simulink model "gm_IP_Core_SS_Switch_and_PWM"  (R2021a)
settings: Solver=VariableStepAuto  StartTime=0.0  StopTime=0.001  RelTol=1e-3
undefined symbols (not defined in the file or in its folder): f_FPGA_clk, T_FPGA_clk
libraries: hdlmdlgenlib x3, hdlsllib x3, simulink x2
(part 3 of 3)

== system gm_IP_Core_SS_Switch_and_PWM/PWM_and_Switching_Signal_Control/GenPWM/Triangle shift1/Subsystem1 ==
  standardized peak of triangle : Inport  OutDataTypeStr=fixdt(0, 21, 17)  PortDimensions=1  SampleTime=1e-08
  triangle_in : Inport  Port=2  OutDataTypeStr=fixdt(1, 20, 17)  PortDimensions=1  SampleTime=1e-08
  converted triangle_shift : Inport  Port=3  OutDataTypeStr=fixdt(1, 20, 17)  PortDimensions=1  SampleTime=1e-08
  modified triangle_shift : Inport  Port=4  OutDataTypeStr=fixdt(1, 20, 17)  PortDimensions=1  SampleTime=1e-08
  Zero_input : Inport  Port=5  OutDataTypeStr=boolean  PortDimensions=1  SampleTime=1e-08
  direction up : Inport  Port=6  OutDataTypeStr=boolean  PortDimensions=1  SampleTime=1e-08
  Relational Operator2 : RelationalOperator  OutDataTypeStr=boolean  SampleTime=1e-08  RndMeth=Nearest
  Sum11_stage2 : Sum  AccumDataTypeStr=fixdt(1, 24, 17)  OutDataTypeStr=fixdt(1, 24, 17)  SampleTime=1e-08
  Sum11_stage3 : Sum  Inputs=+-  AccumDataTypeStr=fixdt(1, 24, 17)  OutDataTypeStr=fixdt(1, 21, 17)  SampleTime=1e-08
  Sum6 : Sum  AccumDataTypeStr=fixdt(1, 23, 17)  OutDataTypeStr=fixdt(1, 23, 17)  SampleTime=1e-08
  and1_1 : Switch  Criteria=u2 > Threshold  Threshold=double(0)  OutDataTypeStr=boolean  SampleTime=1e-08
  and1_2 : Switch  Criteria=u2 > Threshold  Threshold=double(0)  OutDataTypeStr=boolean  SampleTime=1e-08
  delayMatch{,1..3} (4 alike) : Delay  DelayLength=double(1)  InitialCondition=0  SampleTime=1e-08
  shifted triangle_in signal : Outport  SampleTime=1e-08
  enable_out : Outport  Port=2  SampleTime=1e-08
  wires:
  delayMatch/1 -> Sum6/2
  delayMatch2/1 -> and1_1/3
  Relational Operator2/1 -> and1_1/2
  Sum11_stage3/1 -> shifted triangle_in signal/1
  Sum6/1 -> Sum11_stage2/2, Relational Operator2/2
  and1_1/1 -> and1_2/1
  and1_2/1 -> enable_out/1
  Sum11_stage2/1 -> Sum11_stage3/1
  standardized peak of triangle/1 -> delayMatch1/1, delayMatch/1
  triangle_in/1 -> Sum11_stage3/2, Relational Operator2/1
  converted triangle_shift/1 -> and1_1/1
  modified triangle_shift/1 -> Sum6/1
  Zero_input/1 -> delayMatch3/1, delayMatch2/1
  direction up/1 -> and1_2/2
  delayMatch1/1 -> Sum11_stage2/1
  delayMatch3/1 -> and1_2/3

== system gm_IP_Core_SS_Switch_and_PWM/PWM_and_Switching_Signal_Control/GenPWM/Triangle shift1/Subsystem2 ==
  triangle_in : Inport  OutDataTypeStr=fixdt(1, 20, 17)  PortDimensions=1  SampleTime=1e-08
  modified triangle_shift : Inport  Port=2  OutDataTypeStr=fixdt(1, 20, 17)  PortDimensions=1  SampleTime=1e-08
  standardized peak of triangle : Inport  Port=3  OutDataTypeStr=fixdt(0, 21, 17)  PortDimensions=1  SampleTime=1e-08
  Zero_input : Inport  Port=4  OutDataTypeStr=boolean  PortDimensions=1  SampleTime=1e-08
  direction down : Inport  Port=5  OutDataTypeStr=boolean  PortDimensions=1  SampleTime=1e-08
  Relational Operator9 : RelationalOperator  OutDataTypeStr=boolean  SampleTime=1e-08  RndMeth=Nearest
  Sum1 : Sum  Inputs=+-  AccumDataTypeStr=fixdt(1, 23, 17)  OutDataTypeStr=fixdt(1, 23, 17)  SampleTime=1e-08
  Sum5_stage2 : Sum  AccumDataTypeStr=fixdt(1, 24, 17)  OutDataTypeStr=fixdt(1, 24, 17)  SampleTime=1e-08
  Sum5_stage3 : Sum  Inputs=+-  AccumDataTypeStr=fixdt(1, 24, 17)  OutDataTypeStr=fixdt(1, 21, 17)  SampleTime=1e-08
  and : Switch  Criteria=u2 > Threshold  Threshold=double(0)  OutDataTypeStr=boolean  SampleTime=1e-08
  delayMatch : Delay  DelayLength=double(1)  InitialCondition=0  SampleTime=1e-08
  delayMatch1 : Delay  DelayLength=double(1)  InitialCondition=0  SampleTime=1e-08
  delayMatch2 : Delay  DelayLength=double(1)  InitialCondition=0  SampleTime=1e-08
  shifted triangle_in signal : Outport  SampleTime=1e-08
  enable_out : Outport  Port=2  SampleTime=1e-08
  wires:
  delayMatch/1 -> Sum1/1
  delayMatch2/1 -> and/3
  Relational Operator9/1 -> and/1
  Sum1/1 -> Sum5_stage2/1, Relational Operator9/2
  Sum5_stage3/1 -> shifted triangle_in signal/1
  and/1 -> enable_out/1
  Sum5_stage2/1 -> Sum5_stage3/1
  triangle_in/1 -> Sum5_stage3/2, Relational Operator9/1
  modified triangle_shift/1 -> Sum1/2
  standardized peak of triangle/1 -> delayMatch1/1, delayMatch/1
  Zero_input/1 -> delayMatch2/1
  direction down/1 -> and/2
  delayMatch1/1 -> Sum5_stage2/2

== system gm_IP_Core_SS_Switch_and_PWM/PWM_and_Switching_Signal_Control/GenPWM/Triangle shift1/Subsystem3 ==
  triangle_in : Inport  OutDataTypeStr=fixdt(1, 20, 17)  PortDimensions=1  SampleTime=1e-08
  modified triangle_shift : Inport  Port=2  OutDataTypeStr=fixdt(1, 20, 17)  PortDimensions=1  SampleTime=1e-08
  direction up : Inport  Port=3  OutDataTypeStr=boolean  PortDimensions=1  SampleTime=1e-08
  Relational Operator6 : RelationalOperator  Operator=<=  OutDataTypeStr=boolean  SampleTime=1e-08  RndMeth=Nearest
  Sum2 : Sum  Inputs=+-  AccumDataTypeStr=fixdt(1, 21, 17)  OutDataTypeStr=fixdt(1, 21, 17)  SampleTime=1e-08
  Sum3 : Sum  Inputs=+-  AccumDataTypeStr=fixdt(1, 21, 17)  OutDataTypeStr=fixdt(1, 21, 17)  SampleTime=1e-08
  Sum4 : Sum  AccumDataTypeStr=fixdt(1, 21, 17)  OutDataTypeStr=fixdt(1, 21, 17)  SampleTime=1e-08
  Switch3 : Switch  Criteria=u2 > Threshold  Threshold=double(0)  OutDataTypeStr=fixdt(1, 21, 17)  SampleTime=1e-08
  sw : Switch  Criteria=u2 > Threshold  Threshold=double(0)  OutDataTypeStr=fixdt(1, 21, 17)  SampleTime=1e-08
  shifted triangle_in signal : Outport  SampleTime=1e-08
  wires:
  Relational Operator6/1 -> Switch3/2
  Sum2/1 -> Switch3/1
  Sum3/1 -> Switch3/3
  Sum4/1 -> sw/3
  Switch3/1 -> sw/1
  sw/1 -> shifted triangle_in signal/1
  triangle_in/1 -> Sum4/2, Sum3/1, Sum2/2, Relational Operator6/1
  modified triangle_shift/1 -> Sum4/1, Sum3/2, Sum2/1, Relational Operator6/2
  direction up/1 -> sw/2

== system gm_IP_Core_SS_Switch_and_PWM/PWM_and_Switching_Signal_Control/GenPWM/Triangle shift2/Subsystem ==
  Zero_input : Inport  OutDataTypeStr=boolean  PortDimensions=1  SampleTime=1e-08
  converted triangle_shift : Inport  Port=2  OutDataTypeStr=fixdt(1, 20, 17)  PortDimensions=1  SampleTime=1e-08
  modified triangle_shift : Inport  Port=3  OutDataTypeStr=fixdt(1, 20, 17)  PortDimensions=1  SampleTime=1e-08
  triangle_in : Inport  Port=4  OutDataTypeStr=fixdt(1, 20, 17)  PortDimensions=1  SampleTime=1e-08
  direction down : Inport  Port=5  OutDataTypeStr=boolean  PortDimensions=1  SampleTime=1e-08
  Relational Operator11 : RelationalOperator  Operator=<=  OutDataTypeStr=boolean  SampleTime=1e-08  RndMeth=Nearest
  Sum8 : Sum  Inputs=+-  AccumDataTypeStr=fixdt(1, 21, 17)  OutDataTypeStr=fixdt(1, 21, 17)  SampleTime=1e-08
  Unary Minus : UnaryMinus  SampleTime=1e-08
  and2_1 : Switch  Criteria=u2 > Threshold  Threshold=double(0)  OutDataTypeStr=boolean  SampleTime=1e-08
  and2_2 : Switch  Criteria=u2 > Threshold  Threshold=double(0)  OutDataTypeStr=boolean  SampleTime=1e-08
  delayMatch : Delay  DelayLength=double(1)  InitialCondition=0  SampleTime=1e-08
  delayMatch1 : Delay  DelayLength=double(1)  InitialCondition=0  SampleTime=1e-08
  shifted triangle_in signal : Outport  SampleTime=1e-08
  enable_out : Outport  Port=2  SampleTime=1e-08
  wires:
  delayMatch/1 -> and2_1/3
  Relational Operator11/1 -> and2_1/2
  Sum8/1 -> shifted triangle_in signal/1
  Unary Minus/1 -> Sum8/1, Relational Operator11/2
  and2_1/1 -> and2_2/1
  and2_2/1 -> enable_out/1
  Zero_input/1 -> delayMatch1/1, delayMatch/1
  converted triangle_shift/1 -> and2_1/1
  modified triangle_shift/1 -> Unary Minus/1
  triangle_in/1 -> Sum8/2, Relational Operator11/1
  direction down/1 -> and2_2/2
  delayMatch1/1 -> and2_2/3

== system gm_IP_Core_SS_Switch_and_PWM/PWM_and_Switching_Signal_Control/GenPWM/Triangle shift2/Subsystem1 ==
  standardized peak of triangle : Inport  OutDataTypeStr=fixdt(0, 21, 17)  PortDimensions=1  SampleTime=1e-08
  triangle_in : Inport  Port=2  OutDataTypeStr=fixdt(1, 20, 17)  PortDimensions=1  SampleTime=1e-08
  converted triangle_shift : Inport  Port=3  OutDataTypeStr=fixdt(1, 20, 17)  PortDimensions=1  SampleTime=1e-08
  modified triangle_shift : Inport  Port=4  OutDataTypeStr=fixdt(1, 20, 17)  PortDimensions=1  SampleTime=1e-08
  Zero_input : Inport  Port=5  OutDataTypeStr=boolean  PortDimensions=1  SampleTime=1e-08
  direction up : Inport  Port=6  OutDataTypeStr=boolean  PortDimensions=1  SampleTime=1e-08
  Relational Operator2 : RelationalOperator  OutDataTypeStr=boolean  SampleTime=1e-08  RndMeth=Nearest
  Sum11_stage2 : Sum  AccumDataTypeStr=fixdt(1, 24, 17)  OutDataTypeStr=fixdt(1, 24, 17)  SampleTime=1e-08
  Sum11_stage3 : Sum  Inputs=+-  AccumDataTypeStr=fixdt(1, 24, 17)  OutDataTypeStr=fixdt(1, 21, 17)  SampleTime=1e-08
  Sum6 : Sum  AccumDataTypeStr=fixdt(1, 23, 17)  OutDataTypeStr=fixdt(1, 23, 17)  SampleTime=1e-08
  and1_1 : Switch  Criteria=u2 > Threshold  Threshold=double(0)  OutDataTypeStr=boolean  SampleTime=1e-08
  and1_2 : Switch  Criteria=u2 > Threshold  Threshold=double(0)  OutDataTypeStr=boolean  SampleTime=1e-08
  delayMatch{,1..3} (4 alike) : Delay  DelayLength=double(1)  InitialCondition=0  SampleTime=1e-08
  shifted triangle_in signal : Outport  SampleTime=1e-08
  enable_out : Outport  Port=2  SampleTime=1e-08
  wires:
  delayMatch/1 -> Sum6/2
  delayMatch2/1 -> and1_1/3
  Relational Operator2/1 -> and1_1/2
  Sum11_stage3/1 -> shifted triangle_in signal/1
  Sum6/1 -> Sum11_stage2/2, Relational Operator2/2
  and1_1/1 -> and1_2/1
  and1_2/1 -> enable_out/1
  Sum11_stage2/1 -> Sum11_stage3/1
  standardized peak of triangle/1 -> delayMatch1/1, delayMatch/1
  triangle_in/1 -> Sum11_stage3/2, Relational Operator2/1
  converted triangle_shift/1 -> and1_1/1
  modified triangle_shift/1 -> Sum6/1
  Zero_input/1 -> delayMatch3/1, delayMatch2/1
  direction up/1 -> and1_2/2
  delayMatch1/1 -> Sum11_stage2/1
  delayMatch3/1 -> and1_2/3

== system gm_IP_Core_SS_Switch_and_PWM/PWM_and_Switching_Signal_Control/GenPWM/Triangle shift2/Subsystem2 ==
  triangle_in : Inport  OutDataTypeStr=fixdt(1, 20, 17)  PortDimensions=1  SampleTime=1e-08
  modified triangle_shift : Inport  Port=2  OutDataTypeStr=fixdt(1, 20, 17)  PortDimensions=1  SampleTime=1e-08
  standardized peak of triangle : Inport  Port=3  OutDataTypeStr=fixdt(0, 21, 17)  PortDimensions=1  SampleTime=1e-08
  Zero_input : Inport  Port=4  OutDataTypeStr=boolean  PortDimensions=1  SampleTime=1e-08
  direction down : Inport  Port=5  OutDataTypeStr=boolean  PortDimensions=1  SampleTime=1e-08
  Relational Operator9 : RelationalOperator  OutDataTypeStr=boolean  SampleTime=1e-08  RndMeth=Nearest
  Sum1 : Sum  Inputs=+-  AccumDataTypeStr=fixdt(1, 23, 17)  OutDataTypeStr=fixdt(1, 23, 17)  SampleTime=1e-08
  Sum5_stage2 : Sum  AccumDataTypeStr=fixdt(1, 24, 17)  OutDataTypeStr=fixdt(1, 24, 17)  SampleTime=1e-08
  Sum5_stage3 : Sum  Inputs=+-  AccumDataTypeStr=fixdt(1, 24, 17)  OutDataTypeStr=fixdt(1, 21, 17)  SampleTime=1e-08
  and : Switch  Criteria=u2 > Threshold  Threshold=double(0)  OutDataTypeStr=boolean  SampleTime=1e-08
  delayMatch : Delay  DelayLength=double(1)  InitialCondition=0  SampleTime=1e-08
  delayMatch1 : Delay  DelayLength=double(1)  InitialCondition=0  SampleTime=1e-08
  delayMatch2 : Delay  DelayLength=double(1)  InitialCondition=0  SampleTime=1e-08
  shifted triangle_in signal : Outport  SampleTime=1e-08
  enable_out : Outport  Port=2  SampleTime=1e-08
  wires:
  delayMatch/1 -> Sum1/1
  delayMatch2/1 -> and/3
  Relational Operator9/1 -> and/1
  Sum1/1 -> Sum5_stage2/1, Relational Operator9/2
  Sum5_stage3/1 -> shifted triangle_in signal/1
  and/1 -> enable_out/1
  Sum5_stage2/1 -> Sum5_stage3/1
  triangle_in/1 -> Sum5_stage3/2, Relational Operator9/1
  modified triangle_shift/1 -> Sum1/2
  standardized peak of triangle/1 -> delayMatch1/1, delayMatch/1
  Zero_input/1 -> delayMatch2/1
  direction down/1 -> and/2
  delayMatch1/1 -> Sum5_stage2/2

== system gm_IP_Core_SS_Switch_and_PWM/PWM_and_Switching_Signal_Control/GenPWM/Triangle shift2/Subsystem3 ==
  triangle_in : Inport  OutDataTypeStr=fixdt(1, 20, 17)  PortDimensions=1  SampleTime=1e-08
  modified triangle_shift : Inport  Port=2  OutDataTypeStr=fixdt(1, 20, 17)  PortDimensions=1  SampleTime=1e-08
  direction up : Inport  Port=3  OutDataTypeStr=boolean  PortDimensions=1  SampleTime=1e-08
  Relational Operator6 : RelationalOperator  Operator=<=  OutDataTypeStr=boolean  SampleTime=1e-08  RndMeth=Nearest
  Sum2 : Sum  Inputs=+-  AccumDataTypeStr=fixdt(1, 21, 17)  OutDataTypeStr=fixdt(1, 21, 17)  SampleTime=1e-08
  Sum3 : Sum  Inputs=+-  AccumDataTypeStr=fixdt(1, 21, 17)  OutDataTypeStr=fixdt(1, 21, 17)  SampleTime=1e-08
  Sum4 : Sum  AccumDataTypeStr=fixdt(1, 21, 17)  OutDataTypeStr=fixdt(1, 21, 17)  SampleTime=1e-08
  Switch3 : Switch  Criteria=u2 > Threshold  Threshold=double(0)  OutDataTypeStr=fixdt(1, 21, 17)  SampleTime=1e-08
  sw : Switch  Criteria=u2 > Threshold  Threshold=double(0)  OutDataTypeStr=fixdt(1, 21, 17)  SampleTime=1e-08
  shifted triangle_in signal : Outport  SampleTime=1e-08
  wires:
  Relational Operator6/1 -> Switch3/2
  Sum2/1 -> Switch3/1
  Sum3/1 -> Switch3/3
  Sum4/1 -> sw/3
  Switch3/1 -> sw/1
  sw/1 -> shifted triangle_in signal/1
  triangle_in/1 -> Sum4/2, Sum3/1, Sum2/2, Relational Operator6/1
  modified triangle_shift/1 -> Sum4/1, Sum3/2, Sum2/1, Relational Operator6/2
  direction up/1 -> sw/2

== system gm_IP_Core_SS_Switch_and_PWM/PWM_and_Switching_Signal_Control1/GenPWM/Triangle shift/Subsystem ==
  note: AND block replaced with
      | switches for better performance
  Zero_input : Inport
  converted triangle_shift : Inport  Port=2
  modified triangle_shift : Inport  Port=3
  triangle_in : Inport  Port=4
  direction down : Inport  Port=5
  Relational Operator11 : RelationalOperator  Operator=<=  OutDataTypeStr=boolean  RndMeth=Nearest
  Sum8 : Sum  Inputs=|-+
  Unary Minus : UnaryMinus
  and2_1 : Switch  Criteria=u2 > Threshold
  and2_2 : Switch  Criteria=u2 > Threshold
  shifted triangle_in signal : Outport
  enable_out : Outport  Port=2
  wires:
  modified triangle_shift/1 -> Unary Minus/1
  and2_2/1 -> enable_out/1
  converted triangle_shift/1 -> and2_1/1
  triangle_in/1 -> Relational Operator11/1, Sum8/1
  Unary Minus/1 -> Relational Operator11/2, Sum8/2
  Sum8/1 -> shifted triangle_in signal/1
  and2_1/1 -> and2_2/1
  Relational Operator11/1 -> and2_1/2
  Zero_input/1 -> and2_2/3, and2_1/3
  direction down/1 -> and2_2/2

== system gm_IP_Core_SS_Switch_and_PWM/PWM_and_Switching_Signal_Control1/GenPWM/Triangle shift/Subsystem1 ==
  note: AND block replaced with
      | switches for better performance
  note: AND block replaced with
      | switches for better performance
  standardized peak of triangle : Inport
  triangle_in : Inport  Port=2
  converted triangle_shift : Inport  Port=3
  modified triangle_shift : Inport  Port=4
  Zero_input : Inport  Port=5
  direction up : Inport  Port=6
  Relational Operator2 : RelationalOperator  OutDataTypeStr=boolean  RndMeth=Nearest
  Sum11 : Sum  Inputs=++-  OutDataTypeStr=fixdt(1,21,17)
  Sum6 : Sum  Inputs=++|
  and1_1 : Switch  Criteria=u2 > Threshold
  and1_2 : Switch  Criteria=u2 > Threshold
  shifted triangle_in signal : Outport
  enable_out : Outport  Port=2
  wires:
  modified triangle_shift/1 -> Sum6/1
  triangle_in/1 -> Sum11/3, Relational Operator2/1
  direction up/1 -> and1_2/2
  converted triangle_shift/1 -> and1_1/1
  and1_2/1 -> enable_out/1
  standardized peak of triangle/1 -> Sum11/1, Sum6/2
  Zero_input/1 -> and1_1/3, and1_2/3
  Relational Operator2/1 -> and1_1/2
  and1_1/1 -> and1_2/1
  Sum6/1 -> Sum11/2, Relational Operator2/2
  Sum11/1 -> shifted triangle_in signal/1

== system gm_IP_Core_SS_Switch_and_PWM/PWM_and_Switching_Signal_Control1/GenPWM/Triangle shift/Subsystem2 ==
  triangle_in : Inport
  modified triangle_shift : Inport  Port=2
  standardized peak of triangle : Inport  Port=3
  Zero_input : Inport  Port=4
  direction down : Inport  Port=5
  Relational Operator9 : RelationalOperator  OutDataTypeStr=boolean  RndMeth=Nearest
  Sum1 : Sum  Inputs=|-+
  Sum5 : Sum  Inputs=++-  OutDataTypeStr=fixdt(1,21,17)
  and : Switch  Criteria=u2 > Threshold
  shifted triangle_in signal : Outport
  enable_out : Outport  Port=2
  wires:
  modified triangle_shift/1 -> Sum1/1
  Sum5/1 -> shifted triangle_in signal/1
  triangle_in/1 -> Sum5/3, Relational Operator9/1
  and/1 -> enable_out/1
  direction down/1 -> and/2
  Relational Operator9/1 -> and/1
  Sum1/1 -> Sum5/1, Relational Operator9/2
  Zero_input/1 -> and/3
  standardized peak of triangle/1 -> Sum5/2, Sum1/2

== system gm_IP_Core_SS_Switch_and_PWM/PWM_and_Switching_Signal_Control1/GenPWM/Triangle shift/Subsystem3 ==
  triangle_in : Inport
  modified triangle_shift : Inport  Port=2
  direction up : Inport  Port=3
  Relational Operator6 : RelationalOperator  Operator=<=  OutDataTypeStr=boolean  RndMeth=Nearest
  Sum2 : Sum  Inputs=|-+
  Sum3 : Sum  Inputs=|+-
  Sum4 : Sum  Inputs=|++
  Switch3 : Switch  Criteria=u2 > Threshold
  sw : Switch  Criteria=u2 > Threshold
  shifted triangle_in signal : Outport
  wires:
  triangle_in/1 -> Sum4/2, Sum2/1, Sum3/1, Relational Operator6/1
  direction up/1 -> sw/2
  Relational Operator6/1 -> Switch3/2
  sw/1 -> shifted triangle_in signal/1
  Sum2/1 -> Switch3/1
  Sum3/1 -> Switch3/3
  Switch3/1 -> sw/1
  modified triangle_shift/1 -> Relational Operator6/2, Sum2/2, Sum3/2, Sum4/1
  Sum4/1 -> sw/3

== system gm_IP_Core_SS_Switch_and_PWM/PWM_and_Switching_Signal_Control1/GenPWM/Triangle shift1/Subsystem ==
  note: AND block replaced with
      | switches for better performance
  Zero_input : Inport
  converted triangle_shift : Inport  Port=2
  modified triangle_shift : Inport  Port=3
  triangle_in : Inport  Port=4
  direction down : Inport  Port=5
  Relational Operator11 : RelationalOperator  Operator=<=  OutDataTypeStr=boolean  RndMeth=Nearest
  Sum8 : Sum  Inputs=|-+
  Unary Minus : UnaryMinus
  and2_1 : Switch  Criteria=u2 > Threshold
  and2_2 : Switch  Criteria=u2 > Threshold
  shifted triangle_in signal : Outport
  enable_out : Outport  Port=2
  wires:
  modified triangle_shift/1 -> Unary Minus/1
  and2_2/1 -> enable_out/1
  converted triangle_shift/1 -> and2_1/1
  triangle_in/1 -> Relational Operator11/1, Sum8/1
  Unary Minus/1 -> Relational Operator11/2, Sum8/2
  Sum8/1 -> shifted triangle_in signal/1
  and2_1/1 -> and2_2/1
  Relational Operator11/1 -> and2_1/2
  Zero_input/1 -> and2_2/3, and2_1/3
  direction down/1 -> and2_2/2

== system gm_IP_Core_SS_Switch_and_PWM/PWM_and_Switching_Signal_Control1/GenPWM/Triangle shift1/Subsystem1 ==
  note: AND block replaced with
      | switches for better performance
  note: AND block replaced with
      | switches for better performance
  standardized peak of triangle : Inport
  triangle_in : Inport  Port=2
  converted triangle_shift : Inport  Port=3
  modified triangle_shift : Inport  Port=4
  Zero_input : Inport  Port=5
  direction up : Inport  Port=6
  Relational Operator2 : RelationalOperator  OutDataTypeStr=boolean  RndMeth=Nearest
  Sum11 : Sum  Inputs=++-  OutDataTypeStr=fixdt(1,21,17)
  Sum6 : Sum  Inputs=++|
  and1_1 : Switch  Criteria=u2 > Threshold
  and1_2 : Switch  Criteria=u2 > Threshold
  shifted triangle_in signal : Outport
  enable_out : Outport  Port=2
  wires:
  modified triangle_shift/1 -> Sum6/1
  triangle_in/1 -> Sum11/3, Relational Operator2/1
  direction up/1 -> and1_2/2
  converted triangle_shift/1 -> and1_1/1
  and1_2/1 -> enable_out/1
  standardized peak of triangle/1 -> Sum11/1, Sum6/2
  Zero_input/1 -> and1_1/3, and1_2/3
  Relational Operator2/1 -> and1_1/2
  and1_1/1 -> and1_2/1
  Sum6/1 -> Sum11/2, Relational Operator2/2
  Sum11/1 -> shifted triangle_in signal/1

== system gm_IP_Core_SS_Switch_and_PWM/PWM_and_Switching_Signal_Control1/GenPWM/Triangle shift1/Subsystem2 ==
  triangle_in : Inport
  modified triangle_shift : Inport  Port=2
  standardized peak of triangle : Inport  Port=3
  Zero_input : Inport  Port=4
  direction down : Inport  Port=5
  Relational Operator9 : RelationalOperator  OutDataTypeStr=boolean  RndMeth=Nearest
  Sum1 : Sum  Inputs=|-+
  Sum5 : Sum  Inputs=++-  OutDataTypeStr=fixdt(1,21,17)
  and : Switch  Criteria=u2 > Threshold
  shifted triangle_in signal : Outport
  enable_out : Outport  Port=2
  wires:
  modified triangle_shift/1 -> Sum1/1
  Sum5/1 -> shifted triangle_in signal/1
  triangle_in/1 -> Sum5/3, Relational Operator9/1
  and/1 -> enable_out/1
  direction down/1 -> and/2
  Relational Operator9/1 -> and/1
  Sum1/1 -> Sum5/1, Relational Operator9/2
  Zero_input/1 -> and/3
  standardized peak of triangle/1 -> Sum5/2, Sum1/2

== system gm_IP_Core_SS_Switch_and_PWM/PWM_and_Switching_Signal_Control1/GenPWM/Triangle shift1/Subsystem3 ==
  triangle_in : Inport
  modified triangle_shift : Inport  Port=2
  direction up : Inport  Port=3
  Relational Operator6 : RelationalOperator  Operator=<=  OutDataTypeStr=boolean  RndMeth=Nearest
  Sum2 : Sum  Inputs=|-+
  Sum3 : Sum  Inputs=|+-
  Sum4 : Sum  Inputs=|++
  Switch3 : Switch  Criteria=u2 > Threshold
  sw : Switch  Criteria=u2 > Threshold
  shifted triangle_in signal : Outport
  wires:
  triangle_in/1 -> Sum4/2, Sum2/1, Sum3/1, Relational Operator6/1
  direction up/1 -> sw/2
  Relational Operator6/1 -> Switch3/2
  sw/1 -> shifted triangle_in signal/1
  Sum2/1 -> Switch3/1
  Sum3/1 -> Switch3/3
  Switch3/1 -> sw/1
  modified triangle_shift/1 -> Relational Operator6/2, Sum2/2, Sum3/2, Sum4/1
  Sum4/1 -> sw/3

== system gm_IP_Core_SS_Switch_and_PWM/PWM_and_Switching_Signal_Control1/GenPWM/Triangle shift2/Subsystem ==
  note: AND block replaced with
      | switches for better performance
  Zero_input : Inport
  converted triangle_shift : Inport  Port=2
  modified triangle_shift : Inport  Port=3
  triangle_in : Inport  Port=4
  direction down : Inport  Port=5
  Relational Operator11 : RelationalOperator  Operator=<=  OutDataTypeStr=boolean  RndMeth=Nearest
  Sum8 : Sum  Inputs=|-+
  Unary Minus : UnaryMinus
  and2_1 : Switch  Criteria=u2 > Threshold
  and2_2 : Switch  Criteria=u2 > Threshold
  shifted triangle_in signal : Outport
  enable_out : Outport  Port=2
  wires:
  modified triangle_shift/1 -> Unary Minus/1
  and2_2/1 -> enable_out/1
  converted triangle_shift/1 -> and2_1/1
  triangle_in/1 -> Relational Operator11/1, Sum8/1
  Unary Minus/1 -> Relational Operator11/2, Sum8/2
  Sum8/1 -> shifted triangle_in signal/1
  and2_1/1 -> and2_2/1
  Relational Operator11/1 -> and2_1/2
  Zero_input/1 -> and2_2/3, and2_1/3
  direction down/1 -> and2_2/2

== system gm_IP_Core_SS_Switch_and_PWM/PWM_and_Switching_Signal_Control1/GenPWM/Triangle shift2/Subsystem1 ==
  note: AND block replaced with
      | switches for better performance
  note: AND block replaced with
      | switches for better performance
  standardized peak of triangle : Inport
  triangle_in : Inport  Port=2
  converted triangle_shift : Inport  Port=3
  modified triangle_shift : Inport  Port=4
  Zero_input : Inport  Port=5
  direction up : Inport  Port=6
  Relational Operator2 : RelationalOperator  OutDataTypeStr=boolean  RndMeth=Nearest
  Sum11 : Sum  Inputs=++-  OutDataTypeStr=fixdt(1,21,17)
  Sum6 : Sum  Inputs=++|
  and1_1 : Switch  Criteria=u2 > Threshold
  and1_2 : Switch  Criteria=u2 > Threshold
  shifted triangle_in signal : Outport
  enable_out : Outport  Port=2
  wires:
  modified triangle_shift/1 -> Sum6/1
  triangle_in/1 -> Sum11/3, Relational Operator2/1
  direction up/1 -> and1_2/2
  converted triangle_shift/1 -> and1_1/1
  and1_2/1 -> enable_out/1
  standardized peak of triangle/1 -> Sum11/1, Sum6/2
  Zero_input/1 -> and1_1/3, and1_2/3
  Relational Operator2/1 -> and1_1/2
  and1_1/1 -> and1_2/1
  Sum6/1 -> Sum11/2, Relational Operator2/2
  Sum11/1 -> shifted triangle_in signal/1

== system gm_IP_Core_SS_Switch_and_PWM/PWM_and_Switching_Signal_Control1/GenPWM/Triangle shift2/Subsystem2 ==
  triangle_in : Inport
  modified triangle_shift : Inport  Port=2
  standardized peak of triangle : Inport  Port=3
  Zero_input : Inport  Port=4
  direction down : Inport  Port=5
  Relational Operator9 : RelationalOperator  OutDataTypeStr=boolean  RndMeth=Nearest
  Sum1 : Sum  Inputs=|-+
  Sum5 : Sum  Inputs=++-  OutDataTypeStr=fixdt(1,21,17)
  and : Switch  Criteria=u2 > Threshold
  shifted triangle_in signal : Outport
  enable_out : Outport  Port=2
  wires:
  modified triangle_shift/1 -> Sum1/1
  Sum5/1 -> shifted triangle_in signal/1
  triangle_in/1 -> Sum5/3, Relational Operator9/1
  and/1 -> enable_out/1
  direction down/1 -> and/2
  Relational Operator9/1 -> and/1
  Sum1/1 -> Sum5/1, Relational Operator9/2
  Zero_input/1 -> and/3
  standardized peak of triangle/1 -> Sum5/2, Sum1/2

== system gm_IP_Core_SS_Switch_and_PWM/PWM_and_Switching_Signal_Control1/GenPWM/Triangle shift2/Subsystem3 ==
  triangle_in : Inport
  modified triangle_shift : Inport  Port=2
  direction up : Inport  Port=3
  Relational Operator6 : RelationalOperator  Operator=<=  OutDataTypeStr=boolean  RndMeth=Nearest
  Sum2 : Sum  Inputs=|-+
  Sum3 : Sum  Inputs=|+-
  Sum4 : Sum  Inputs=|++
  Switch3 : Switch  Criteria=u2 > Threshold
  sw : Switch  Criteria=u2 > Threshold
  shifted triangle_in signal : Outport
  wires:
  triangle_in/1 -> Sum4/2, Sum2/1, Sum3/1, Relational Operator6/1
  direction up/1 -> sw/2
  Relational Operator6/1 -> Switch3/2
  sw/1 -> shifted triangle_in signal/1
  Sum2/1 -> Switch3/1
  Sum3/1 -> Switch3/3
  Switch3/1 -> sw/1
  modified triangle_shift/1 -> Relational Operator6/2, Sum2/2, Sum3/2, Sum4/1
  Sum4/1 -> sw/3
